simulink model "feedback_plant"  (R2016a)
settings: Solver=ode14x  StartTime=0.0  StopTime=inf  FixedStep=T_sample_control  MaxStep=0.1  RelTol=1e-3
undefined symbols (not defined in the file): b, J, K, L, R
libraries: simulink x1
settings Model: ModifiedByFormat=The MathWorks Inc.  Creator=The MathWorks, Inc.  LastModifiedBy=The MathWorks Inc.
settings DataIOCC: SaveFormat=Array
settings OptimizationCC: DefaultParameterBehavior=Inlined  ExpressionDepthLimit=2147483647
settings DebuggingCC: UnderspecifiedInitializationDetection=Classic  MergeDetectMultiDrivingBlocksExec=none  SolverPrmCheckMsg=warning  FcnCallInpInsideContextMsg=EnableAllAsWarning  RootOutportRequireBusObject=error  AllowSymbolicDim=off  StateNameClashWarn=warning  StrictBusMsg=ErrorOnBusTreatedAsVector
settings HardwareCC: ProdBitPerPointer=32  ProdLargestAtomicFloat=None  ProdWordSize=32  ProdHWDeviceType=Intel->x86/Pentium
settings ModelReferenceCC: PropagateSignalLabelsOutOfModel=off
settings RTWCC: SystemTargetFile=NIVeriStand.tlc  TemplateMakefile=NIVeriStand_vc.tmf  Description=NI Phar Lap Real-Time & Windows Targets
settings STFCustomTargetCC: MatFileLogging=on  MATLABClassNameForMDSCustomization=Simulink.SoftwareTarget.TargetSpecificTriggerConfigurationBase  SystemTargetFile=NIVeriStand.tlc
settings ConfigComp: CovModelRefEnable=Off  CovSFcnEnable=off

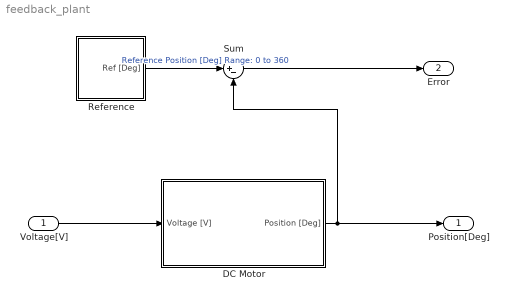
== system feedback_plant ==
  Voltage[V] : Inport
  DC Motor : Subsystem
  Reference : Subsystem
  Sum : Sum  Inputs=|+-
  Position[Deg] : Outport
  Error : Outport  Port=2
  wires:
  Voltage[V]/1 -> DC Motor/1(Voltage [V])
  DC Motor/1(Position [Deg]) -> Position[Deg]/1, Sum/2
  Reference/1(Ref [Deg]) -> Sum/1  "Reference Position [Deg] Range: 0 to 360"
  Sum/1 -> Error/1

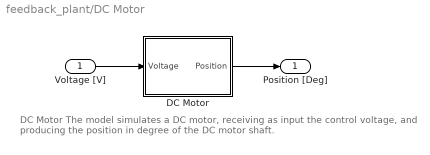
== system feedback_plant/DC Motor ==
  note: DC Motor
      | The model simulates a DC motor, receiving as input the control voltage, and producing the position in degree of the DC motor shaft.
  Voltage [V] : Inport
  DC Motor : Subsystem
  Position [Deg] : Outport
  wires:
  Voltage [V]/1 -> DC Motor/1(Voltage)
  DC Motor/1(Position) -> Position [Deg]/1

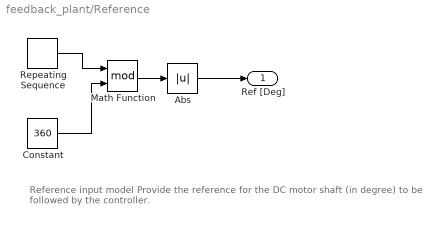
== system feedback_plant/Reference ==
  note: Reference input model
      | Provide the reference for the DC motor shaft (in degree) to be followed by the controller.
  Abs : Abs
  Constant : Constant  Value=360
  Math Function : Math  Operator=mod  SaturateOnIntegerOverflow=on
  Repeating Sequence : simulink/Sources/Repeating Sequence  rep_seq_t=[0 0.1 2 2.1 4]  rep_seq_y=[0 88 88 0 0].'
  Ref [Deg] : Outport
  wires:
  Constant/1 -> Math Function/2
  Repeating Sequence/1 -> Math Function/1
  Math Function/1 -> Abs/1
  Abs/1 -> Ref [Deg]/1

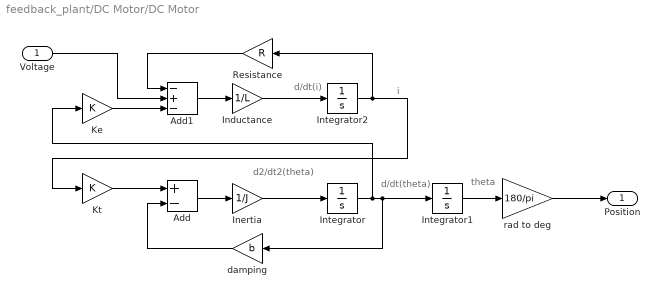
== system feedback_plant/DC Motor/DC Motor ==
  note: i
  note: d/dt(theta)
  note: d2/dt2(theta)
  note: d/dt(i)
  note: theta
  Voltage : Inport
  Add : Sum  Inputs=+-
  Add1 : Sum  Inputs=-+-
  Inductance : Gain  Gain=1/L
  Inertia : Gain  Gain=1/J
  Integrator : Integrator
  Integrator1 : Integrator
  Integrator2 : Integrator
  Ke : Gain  Gain=K
  Kt : Gain  Gain=K
  Resistance : Gain  Gain=R
  damping : Gain  Gain=b
  rad to deg : Gain  Gain=180/pi
  Position : Outport
  wires:
  Inductance/1 -> Integrator2/1
  Integrator/1 -> Integrator1/1, damping/1, Ke/1
  Integrator1/1 -> rad to deg/1
  Inertia/1 -> Integrator/1
  Integrator2/1 -> Kt/1, Resistance/1
  Add/1 -> Inertia/1
  Add1/1 -> Inductance/1
  Kt/1 -> Add/1
  damping/1 -> Add/2
  Ke/1 -> Add1/3
  Resistance/1 -> Add1/1
  Voltage/1 -> Add1/2
  rad to deg/1 -> Position/1
